simulink model "quartercar"  (R2013a)
settings: Solver=ode15s  StartTime=0  StopTime=60  RelTol=1e-3
libraries: simulink x3
settings Model: Creator=Administrator  LastModifiedBy=Tran Duc Chung
settings DataIOCC: LimitDataPoints=off

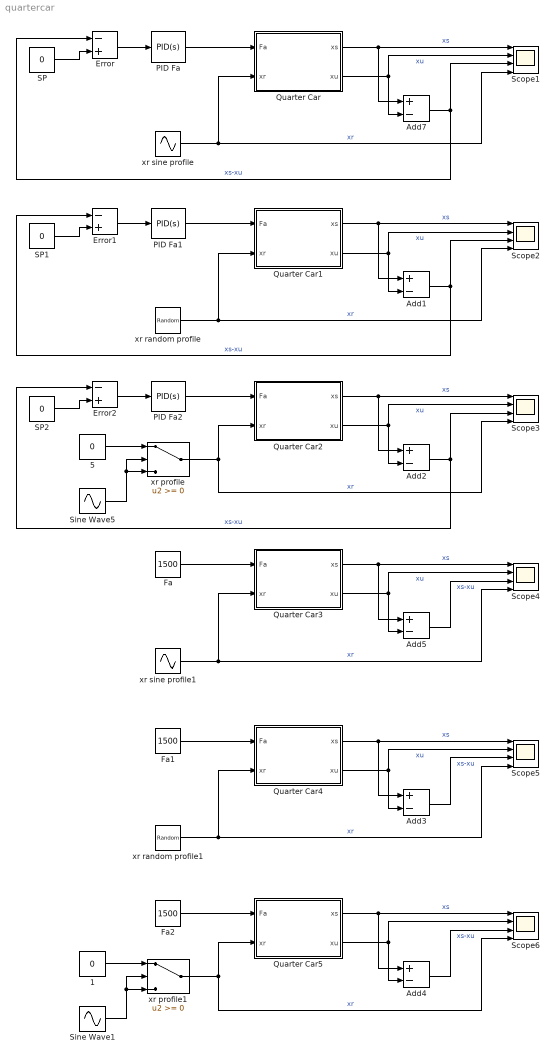
== system quartercar ==
  1 : Constant  Value=0
  5 : Constant  Value=0
  Add{1..5,7} (6 alike) : Sum  Inputs=+-
  Error : Sum  Inputs=-+
  Error1 : Sum  Inputs=-+
  Error2 : Sum  Inputs=-+
  Fa : Constant  Value=1500
  Fa1 : Constant  Value=1500
  Fa2 : Constant  Value=1500
  PID Fa : simulink/Continuous/PID Controller  Controller=PID  TimeDomain=Continuous-time  SampleTime=1  IntegratorMethod=Forward Euler  FilterMethod=Forward Euler  Form=Parallel  P=0  I=17490.1289315124  D=0  N=100  InitialConditionSource=internal  InitialConditionForIntegrator=0  InitialConditionForFilter=0  ExternalReset=none  LimitOutput=on  UpperSaturationLimit=3000  LowerSaturationLimit=0  LinearizeAsGain=on  AntiWindupMode=none  Kb=1  TrackingMode=off  Kt=1  PParamMin=[]  PParamMax=[]  IParamMin=[]  IParamMax=[]  DParamMin=[]  DParamMax=[]  NParamMin=[]  NParamMax=[]  KbParamMin=[]  KbParamMax=[]  KtParamMin=[]  KtParamMax=[]  POutMin=[]  POutMax=[]  IOutMin=[]  IOutMax=[]  DOutMin=[]  DOutMax=[]  NOutMin=[]  NOutMax=[]  KbOutMin=[]  KbOutMax=[]  KtOutMin=[]  KtOutMax=[]  IntegratorOutMin=[]  IntegratorOutMax=[]  FilterOutMin=[]  FilterOutMax=[]  SumOutMin=[]  SumOutMax=[]  SumI1OutMin=[]  SumI1OutMax=[]  SumI2OutMin=[]  SumI2OutMax=[]  SumI3OutMin=[]  SumI3OutMax=[]  SumDOutMin=[]  SumDOutMax=[]  SaturationOutMin=[]  SaturationOutMax=[]  IntegratorContinuousStateAttributes=''  IntegratorStateMustResolveToSignalObject=off  IntegratorRTWStateStorageClass=Auto  FilterContinuousStateAttributes=''  FilterStateMustResolveToSignalObject=off  FilterRTWStateStorageClass=Auto
  PID Fa1 : simulink/Continuous/PID Controller  Controller=PID  TimeDomain=Continuous-time  SampleTime=1  IntegratorMethod=Forward Euler  FilterMethod=Forward Euler  Form=Parallel  P=0  I=17490.1289315124  D=0  N=100  InitialConditionSource=internal  InitialConditionForIntegrator=0  InitialConditionForFilter=0  ExternalReset=none  LimitOutput=on  UpperSaturationLimit=3000  LowerSaturationLimit=0  LinearizeAsGain=on  AntiWindupMode=none  Kb=1  TrackingMode=off  Kt=1  PParamMin=[]  PParamMax=[]  IParamMin=[]  IParamMax=[]  DParamMin=[]  DParamMax=[]  NParamMin=[]  NParamMax=[]  KbParamMin=[]  KbParamMax=[]  KtParamMin=[]  KtParamMax=[]  POutMin=[]  POutMax=[]  IOutMin=[]  IOutMax=[]  DOutMin=[]  DOutMax=[]  NOutMin=[]  NOutMax=[]  KbOutMin=[]  KbOutMax=[]  KtOutMin=[]  KtOutMax=[]  IntegratorOutMin=[]  IntegratorOutMax=[]  FilterOutMin=[]  FilterOutMax=[]  SumOutMin=[]  SumOutMax=[]  SumI1OutMin=[]  SumI1OutMax=[]  SumI2OutMin=[]  SumI2OutMax=[]  SumI3OutMin=[]  SumI3OutMax=[]  SumDOutMin=[]  SumDOutMax=[]  SaturationOutMin=[]  SaturationOutMax=[]  IntegratorContinuousStateAttributes=''  IntegratorStateMustResolveToSignalObject=off  IntegratorRTWStateStorageClass=Auto  FilterContinuousStateAttributes=''  FilterStateMustResolveToSignalObject=off  FilterRTWStateStorageClass=Auto
  PID Fa2 : simulink/Continuous/PID Controller  Controller=PID  TimeDomain=Continuous-time  SampleTime=1  IntegratorMethod=Forward Euler  FilterMethod=Forward Euler  Form=Parallel  P=0  I=17490.1289315124  D=0  N=100  InitialConditionSource=internal  InitialConditionForIntegrator=0  InitialConditionForFilter=0  ExternalReset=none  LimitOutput=on  UpperSaturationLimit=3000  LowerSaturationLimit=0  LinearizeAsGain=on  AntiWindupMode=none  Kb=1  TrackingMode=off  Kt=1  PParamMin=[]  PParamMax=[]  IParamMin=[]  IParamMax=[]  DParamMin=[]  DParamMax=[]  NParamMin=[]  NParamMax=[]  KbParamMin=[]  KbParamMax=[]  KtParamMin=[]  KtParamMax=[]  POutMin=[]  POutMax=[]  IOutMin=[]  IOutMax=[]  DOutMin=[]  DOutMax=[]  NOutMin=[]  NOutMax=[]  KbOutMin=[]  KbOutMax=[]  KtOutMin=[]  KtOutMax=[]  IntegratorOutMin=[]  IntegratorOutMax=[]  FilterOutMin=[]  FilterOutMax=[]  SumOutMin=[]  SumOutMax=[]  SumI1OutMin=[]  SumI1OutMax=[]  SumI2OutMin=[]  SumI2OutMax=[]  SumI3OutMin=[]  SumI3OutMax=[]  SumDOutMin=[]  SumDOutMax=[]  SaturationOutMin=[]  SaturationOutMax=[]  IntegratorContinuousStateAttributes=''  IntegratorStateMustResolveToSignalObject=off  IntegratorRTWStateStorageClass=Auto  FilterContinuousStateAttributes=''  FilterStateMustResolveToSignalObject=off  FilterRTWStateStorageClass=Auto
  Quarter Car : Subsystem
  Quarter Car1 : Subsystem
  Quarter Car2 : Subsystem
  Quarter Car3 : Subsystem
  Quarter Car4 : Subsystem
  Quarter Car5 : Subsystem
  SP : Constant  Value=0
  SP1 : Constant  Value=0
  SP2 : Constant  Value=0
  Scope{1..6} (6 alike) : Scope  NumInputPorts=4
      Scope1 settings: YMin=-5~-5~-5~-5  YMax=5~5~5~5  SaveName=ScopeData3
      Scope2 settings: YMin=-5~-5~-5~-5  YMax=5~5~5~5
      Scope3 settings: YMin=-5~-5~-5~-5  YMax=5~5~5~5
      Scope4 settings: YMin=-5~-5~-5~-5  YMax=5~5~5~5  SaveName=ScopeData2
      Scope5 settings: YMin=-5~-5~-5~-5  YMax=5~5~5~5  SaveName=ScopeData4
      Scope6 settings: YMin=-5~-5~-5~-5  YMax=5~5~5~5  SaveName=ScopeData5
  Sine Wave1 : Sin  Amplitude=0.05  SampleTime=0
  Sine Wave5 : Sin  Amplitude=0.05  SampleTime=0
  xr profile : Switch
  xr profile1 : Switch
  xr random profile : RandomNumber  Variance=0.0005  SampleTime=0.1
  xr random profile1 : RandomNumber  Variance=0.0005  SampleTime=0.1
  xr sine profile : Sin  Amplitude=0.05  SampleTime=0
  xr sine profile1 : Sin  Amplitude=0.05  SampleTime=0
  wires:
  Error/1 -> PID Fa/1
  SP/1 -> Error/2
  5/1 -> xr profile/1
  Sine Wave5/1 -> xr profile/3, xr profile/2
  Quarter Car/1(xs) -> Add7/1, Scope1/1  "xs"
  Quarter Car/2(xu) -> Scope1/2, Add7/2  "xu"
  xr sine profile/1 -> Scope1/4, Quarter Car/2(xr)  "xr"
  PID Fa/1 -> Quarter Car/1(Fa)
  Add7/1 -> Scope1/3, Error/1  "xs-xu"
  Error1/1 -> PID Fa1/1
  SP1/1 -> Error1/2
  Quarter Car1/1(xs) -> Add1/1, Scope2/1  "xs"
  Quarter Car1/2(xu) -> Scope2/2, Add1/2  "xu"
  xr random profile/1 -> Scope2/4, Quarter Car1/2(xr)  "xr"
  PID Fa1/1 -> Quarter Car1/1(Fa)
  Add1/1 -> Scope2/3, Error1/1  "xs-xu"
  Error2/1 -> PID Fa2/1
  SP2/1 -> Error2/2
  Quarter Car2/1(xs) -> Add2/1, Scope3/1  "xs"
  Quarter Car2/2(xu) -> Scope3/2, Add2/2  "xu"
  xr profile/1 -> Scope3/4, Quarter Car2/2(xr)  "xr"
  PID Fa2/1 -> Quarter Car2/1(Fa)
  Add2/1 -> Scope3/3, Error2/1  "xs-xu"
  1/1 -> xr profile1/1
  Sine Wave1/1 -> xr profile1/3, xr profile1/2
  Quarter Car3/1(xs) -> Add5/1, Scope4/1  "xs"
  Quarter Car3/2(xu) -> Scope4/2, Add5/2  "xu"
  xr sine profile1/1 -> Scope4/4, Quarter Car3/2(xr)  "xr"
  Fa/1 -> Quarter Car3/1(Fa)
  Add5/1 -> Scope4/3  "xs-xu"
  Quarter Car4/1(xs) -> Add3/1, Scope5/1  "xs"
  Quarter Car4/2(xu) -> Scope5/2, Add3/2  "xu"
  xr random profile1/1 -> Scope5/4, Quarter Car4/2(xr)  "xr"
  Fa1/1 -> Quarter Car4/1(Fa)
  Add3/1 -> Scope5/3  "xs-xu"
  Quarter Car5/1(xs) -> Add4/1, Scope6/1  "xs"
  Quarter Car5/2(xu) -> Scope6/2, Add4/2
  xr profile1/1 -> Scope6/4, Quarter Car5/2(xr)  "xr"
  Fa2/1 -> Quarter Car5/1(Fa)
  Add4/1 -> Scope6/3  "xs-xu"

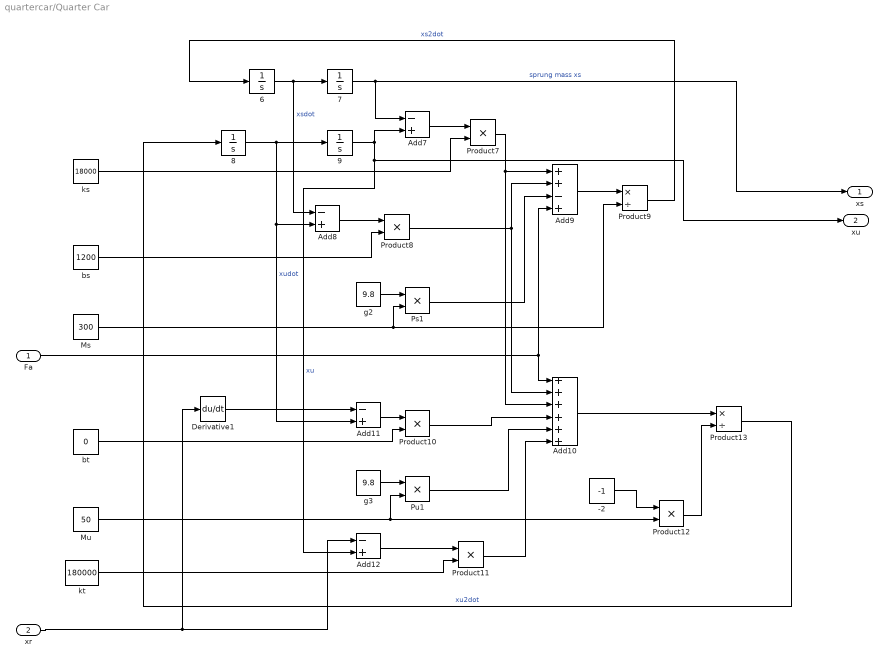
== system quartercar/Quarter Car ==
  Fa : Inport
  xr : Inport  Port=2
  -2 : Constant  Value=-1
  {6..9} (4 alike) : Integrator
  Add10 : Sum  Inputs=++++++
  Add{7..8,11..12} (4 alike) : Sum  Inputs=-+
  Add9 : Sum  Inputs=++-+
  Derivative1 : Derivative
  Ms : Constant  Value=300
  Mu : Constant  Value=50
  Product{7..8,10..12} (5 alike) : Product
  Product13 : Product  Inputs=*/
  Product9 : Product  Inputs=*/
  Ps1 : Product
  Pu1 : Product
  bs : Constant  Value=1200
  bt : Constant  Value=0
  g2 : Constant  Value=9.8
  g3 : Constant  Value=9.8
  ks : Constant  Value=18000
  kt : Constant  Value=180000
  xs : Outport
  xu : Outport  Port=2
  wires:
  g2/1 -> Ps1/1
  Product12/1 -> Product13/2
  g3/1 -> Pu1/1
  Ps1/1 -> Add9/3
  Add10/1 -> Product13/1
  -2/1 -> Product12/1
  Mu/1 -> Pu1/2, Product12/2
  Product11/1 -> Add10/6
  Add12/1 -> Product11/1
  kt/1 -> Product11/2
  xr/1 -> Add12/1, Derivative1/1
  Pu1/1 -> Add10/5
  Product10/1 -> Add10/4
  Add11/1 -> Product10/1
  bt/1 -> Product10/2
  Derivative1/1 -> Add11/1
  Ms/1 -> Product9/2, Ps1/2
  Add9/1 -> Product9/1
  Fa/1 -> Add10/1, Add9/4
  Product8/1 -> Add10/2, Add9/2
  Product7/1 -> Add10/3, Add9/1
  bs/1 -> Product8/2
  Add8/1 -> Product8/1
  ks/1 -> Product7/2
  Add7/1 -> Product7/1
  9/1 -> Add12/2, xu/1, Add7/2  "xu"
  Product13/1 -> 8/1  "xu2dot"
  8/1 -> 9/1, Add8/2, Add11/2  "xudot"
  7/1 -> Add7/1, xs/1  "sprung mass xs"
  Product9/1 -> 6/1  "xs2dot"
  6/1 -> 7/1, Add8/1  "xsdot"

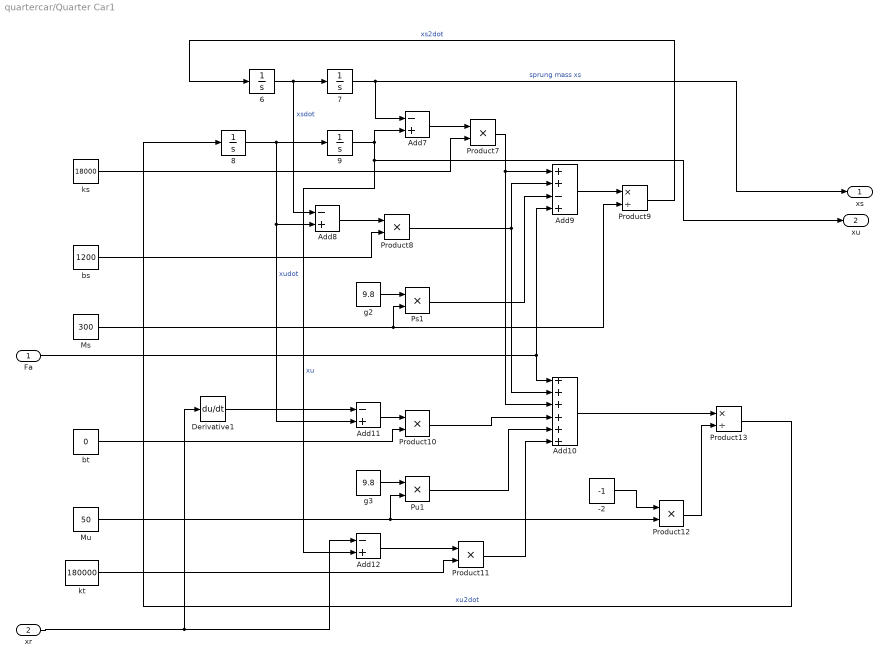
== system quartercar/Quarter Car1 ==
  Fa : Inport
  xr : Inport  Port=2
  -2 : Constant  Value=-1
  {6..9} (4 alike) : Integrator
  Add10 : Sum  Inputs=++++++
  Add{7..8,11..12} (4 alike) : Sum  Inputs=-+
  Add9 : Sum  Inputs=++-+
  Derivative1 : Derivative
  Ms : Constant  Value=300
  Mu : Constant  Value=50
  Product{7..8,10..12} (5 alike) : Product
  Product13 : Product  Inputs=*/
  Product9 : Product  Inputs=*/
  Ps1 : Product
  Pu1 : Product
  bs : Constant  Value=1200
  bt : Constant  Value=0
  g2 : Constant  Value=9.8
  g3 : Constant  Value=9.8
  ks : Constant  Value=18000
  kt : Constant  Value=180000
  xs : Outport
  xu : Outport  Port=2
  wires:
  g2/1 -> Ps1/1
  Product12/1 -> Product13/2
  g3/1 -> Pu1/1
  Ps1/1 -> Add9/3
  Add10/1 -> Product13/1
  -2/1 -> Product12/1
  Mu/1 -> Pu1/2, Product12/2
  Product11/1 -> Add10/6
  Add12/1 -> Product11/1
  kt/1 -> Product11/2
  xr/1 -> Add12/1, Derivative1/1
  Pu1/1 -> Add10/5
  Product10/1 -> Add10/4
  Add11/1 -> Product10/1
  bt/1 -> Product10/2
  Derivative1/1 -> Add11/1
  Ms/1 -> Product9/2, Ps1/2
  Add9/1 -> Product9/1
  Fa/1 -> Add10/1, Add9/4
  Product8/1 -> Add10/2, Add9/2
  Product7/1 -> Add10/3, Add9/1
  bs/1 -> Product8/2
  Add8/1 -> Product8/1
  ks/1 -> Product7/2
  Add7/1 -> Product7/1
  9/1 -> Add12/2, xu/1, Add7/2  "xu"
  Product13/1 -> 8/1  "xu2dot"
  8/1 -> 9/1, Add8/2, Add11/2  "xudot"
  7/1 -> Add7/1, xs/1  "sprung mass xs"
  Product9/1 -> 6/1  "xs2dot"
  6/1 -> 7/1, Add8/1  "xsdot"

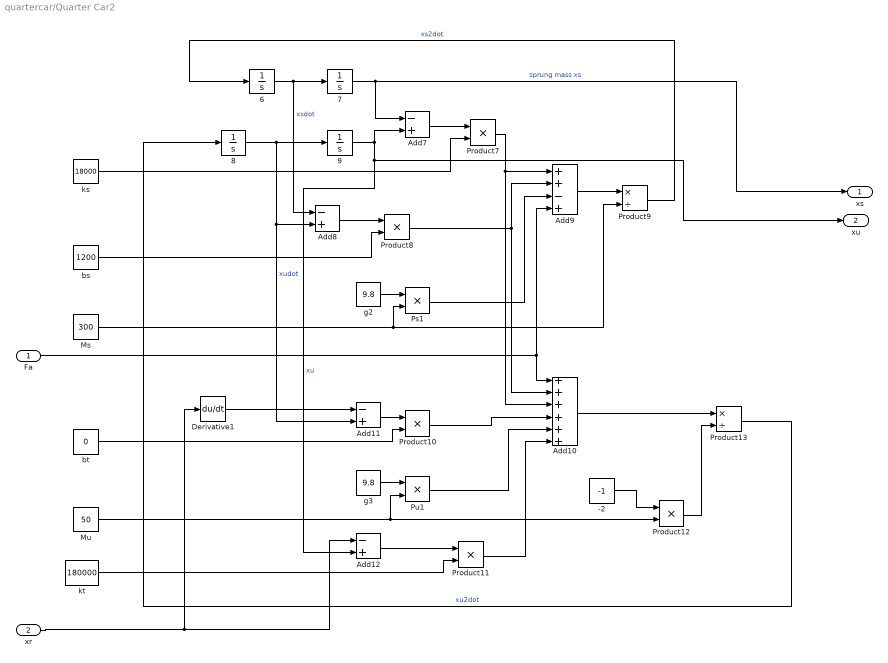
== system quartercar/Quarter Car2 ==
  Fa : Inport
  xr : Inport  Port=2
  -2 : Constant  Value=-1
  {6..9} (4 alike) : Integrator
  Add10 : Sum  Inputs=++++++
  Add{7..8,11..12} (4 alike) : Sum  Inputs=-+
  Add9 : Sum  Inputs=++-+
  Derivative1 : Derivative
  Ms : Constant  Value=300
  Mu : Constant  Value=50
  Product{7..8,10..12} (5 alike) : Product
  Product13 : Product  Inputs=*/
  Product9 : Product  Inputs=*/
  Ps1 : Product
  Pu1 : Product
  bs : Constant  Value=1200
  bt : Constant  Value=0
  g2 : Constant  Value=9.8
  g3 : Constant  Value=9.8
  ks : Constant  Value=18000
  kt : Constant  Value=180000
  xs : Outport
  xu : Outport  Port=2
  wires:
  g2/1 -> Ps1/1
  Product12/1 -> Product13/2
  g3/1 -> Pu1/1
  Ps1/1 -> Add9/3
  Add10/1 -> Product13/1
  -2/1 -> Product12/1
  Mu/1 -> Pu1/2, Product12/2
  Product11/1 -> Add10/6
  Add12/1 -> Product11/1
  kt/1 -> Product11/2
  xr/1 -> Add12/1, Derivative1/1
  Pu1/1 -> Add10/5
  Product10/1 -> Add10/4
  Add11/1 -> Product10/1
  bt/1 -> Product10/2
  Derivative1/1 -> Add11/1
  Ms/1 -> Product9/2, Ps1/2
  Add9/1 -> Product9/1
  Fa/1 -> Add10/1, Add9/4
  Product8/1 -> Add10/2, Add9/2
  Product7/1 -> Add10/3, Add9/1
  bs/1 -> Product8/2
  Add8/1 -> Product8/1
  ks/1 -> Product7/2
  Add7/1 -> Product7/1
  9/1 -> Add12/2, xu/1, Add7/2  "xu"
  Product13/1 -> 8/1  "xu2dot"
  8/1 -> 9/1, Add8/2, Add11/2  "xudot"
  7/1 -> Add7/1, xs/1  "sprung mass xs"
  Product9/1 -> 6/1  "xs2dot"
  6/1 -> 7/1, Add8/1  "xsdot"

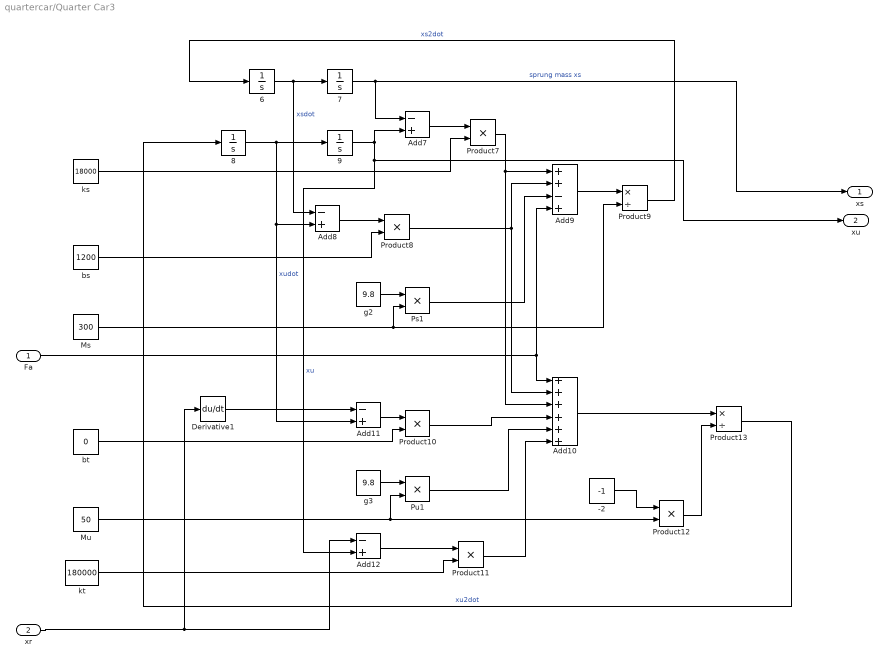
== system quartercar/Quarter Car3 ==
  Fa : Inport
  xr : Inport  Port=2
  -2 : Constant  Value=-1
  {6..9} (4 alike) : Integrator
  Add10 : Sum  Inputs=++++++
  Add{7..8,11..12} (4 alike) : Sum  Inputs=-+
  Add9 : Sum  Inputs=++-+
  Derivative1 : Derivative
  Ms : Constant  Value=300
  Mu : Constant  Value=50
  Product{7..8,10..12} (5 alike) : Product
  Product13 : Product  Inputs=*/
  Product9 : Product  Inputs=*/
  Ps1 : Product
  Pu1 : Product
  bs : Constant  Value=1200
  bt : Constant  Value=0
  g2 : Constant  Value=9.8
  g3 : Constant  Value=9.8
  ks : Constant  Value=18000
  kt : Constant  Value=180000
  xs : Outport
  xu : Outport  Port=2
  wires:
  g2/1 -> Ps1/1
  Product12/1 -> Product13/2
  g3/1 -> Pu1/1
  Ps1/1 -> Add9/3
  Add10/1 -> Product13/1
  -2/1 -> Product12/1
  Mu/1 -> Pu1/2, Product12/2
  Product11/1 -> Add10/6
  Add12/1 -> Product11/1
  kt/1 -> Product11/2
  xr/1 -> Add12/1, Derivative1/1
  Pu1/1 -> Add10/5
  Product10/1 -> Add10/4
  Add11/1 -> Product10/1
  bt/1 -> Product10/2
  Derivative1/1 -> Add11/1
  Ms/1 -> Product9/2, Ps1/2
  Add9/1 -> Product9/1
  Fa/1 -> Add10/1, Add9/4
  Product8/1 -> Add10/2, Add9/2
  Product7/1 -> Add10/3, Add9/1
  bs/1 -> Product8/2
  Add8/1 -> Product8/1
  ks/1 -> Product7/2
  Add7/1 -> Product7/1
  9/1 -> Add12/2, xu/1, Add7/2  "xu"
  Product13/1 -> 8/1  "xu2dot"
  8/1 -> 9/1, Add8/2, Add11/2  "xudot"
  7/1 -> Add7/1, xs/1  "sprung mass xs"
  Product9/1 -> 6/1  "xs2dot"
  6/1 -> 7/1, Add8/1  "xsdot"

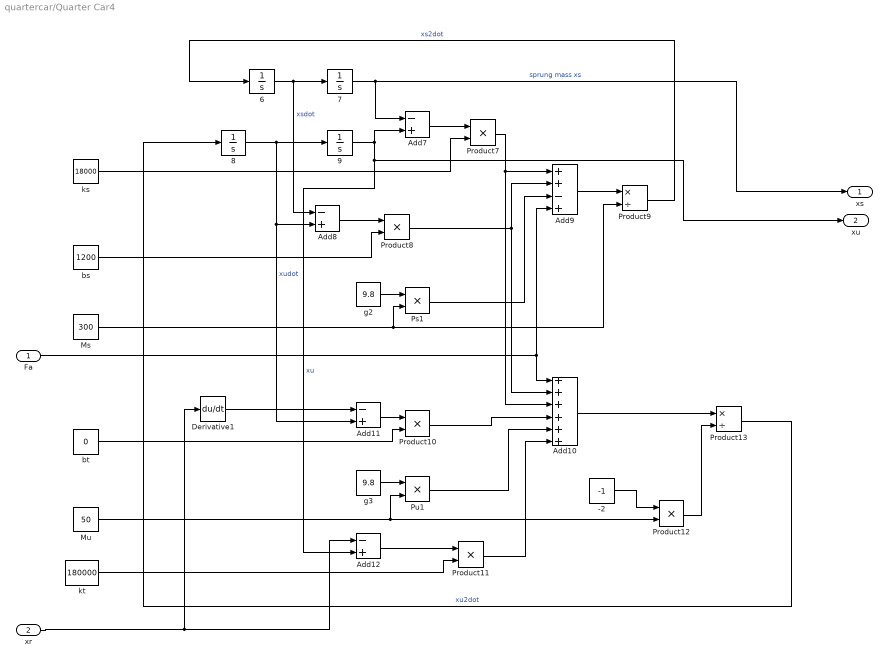
== system quartercar/Quarter Car4 ==
  Fa : Inport
  xr : Inport  Port=2
  -2 : Constant  Value=-1
  {6..9} (4 alike) : Integrator
  Add10 : Sum  Inputs=++++++
  Add{7..8,11..12} (4 alike) : Sum  Inputs=-+
  Add9 : Sum  Inputs=++-+
  Derivative1 : Derivative
  Ms : Constant  Value=300
  Mu : Constant  Value=50
  Product{7..8,10..12} (5 alike) : Product
  Product13 : Product  Inputs=*/
  Product9 : Product  Inputs=*/
  Ps1 : Product
  Pu1 : Product
  bs : Constant  Value=1200
  bt : Constant  Value=0
  g2 : Constant  Value=9.8
  g3 : Constant  Value=9.8
  ks : Constant  Value=18000
  kt : Constant  Value=180000
  xs : Outport
  xu : Outport  Port=2
  wires:
  g2/1 -> Ps1/1
  Product12/1 -> Product13/2
  g3/1 -> Pu1/1
  Ps1/1 -> Add9/3
  Add10/1 -> Product13/1
  -2/1 -> Product12/1
  Mu/1 -> Pu1/2, Product12/2
  Product11/1 -> Add10/6
  Add12/1 -> Product11/1
  kt/1 -> Product11/2
  xr/1 -> Add12/1, Derivative1/1
  Pu1/1 -> Add10/5
  Product10/1 -> Add10/4
  Add11/1 -> Product10/1
  bt/1 -> Product10/2
  Derivative1/1 -> Add11/1
  Ms/1 -> Product9/2, Ps1/2
  Add9/1 -> Product9/1
  Fa/1 -> Add10/1, Add9/4
  Product8/1 -> Add10/2, Add9/2
  Product7/1 -> Add10/3, Add9/1
  bs/1 -> Product8/2
  Add8/1 -> Product8/1
  ks/1 -> Product7/2
  Add7/1 -> Product7/1
  9/1 -> Add12/2, xu/1, Add7/2  "xu"
  Product13/1 -> 8/1  "xu2dot"
  8/1 -> 9/1, Add8/2, Add11/2  "xudot"
  7/1 -> Add7/1, xs/1  "sprung mass xs"
  Product9/1 -> 6/1  "xs2dot"
  6/1 -> 7/1, Add8/1  "xsdot"

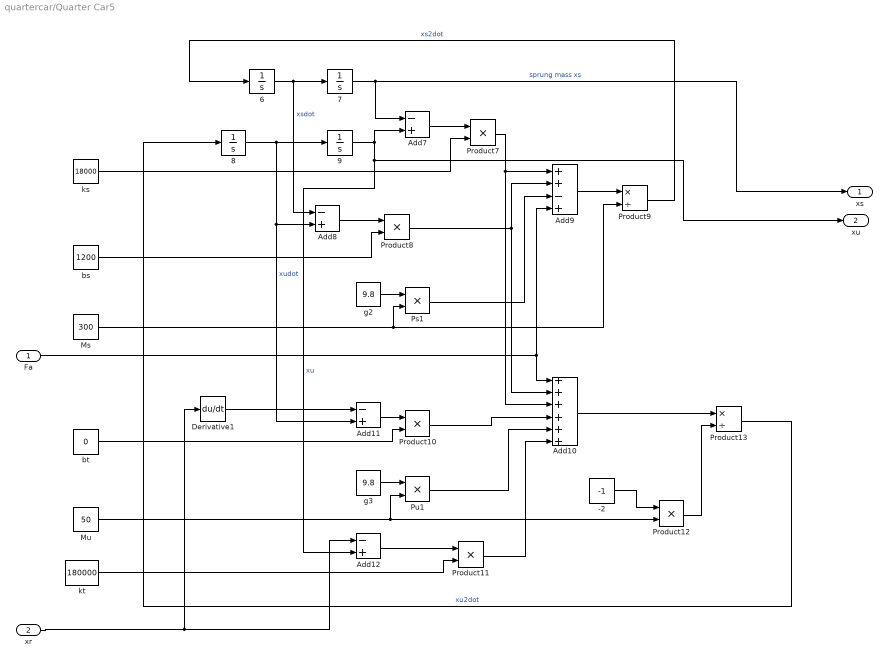
== system quartercar/Quarter Car5 ==
  Fa : Inport
  xr : Inport  Port=2
  -2 : Constant  Value=-1
  {6..9} (4 alike) : Integrator
  Add10 : Sum  Inputs=++++++
  Add{7..8,11..12} (4 alike) : Sum  Inputs=-+
  Add9 : Sum  Inputs=++-+
  Derivative1 : Derivative
  Ms : Constant  Value=300
  Mu : Constant  Value=50
  Product{7..8,10..12} (5 alike) : Product
  Product13 : Product  Inputs=*/
  Product9 : Product  Inputs=*/
  Ps1 : Product
  Pu1 : Product
  bs : Constant  Value=1200
  bt : Constant  Value=0
  g2 : Constant  Value=9.8
  g3 : Constant  Value=9.8
  ks : Constant  Value=18000
  kt : Constant  Value=180000
  xs : Outport
  xu : Outport  Port=2
  wires:
  g2/1 -> Ps1/1
  Product12/1 -> Product13/2
  g3/1 -> Pu1/1
  Ps1/1 -> Add9/3
  Add10/1 -> Product13/1
  -2/1 -> Product12/1
  Mu/1 -> Pu1/2, Product12/2
  Product11/1 -> Add10/6
  Add12/1 -> Product11/1
  kt/1 -> Product11/2
  xr/1 -> Add12/1, Derivative1/1
  Pu1/1 -> Add10/5
  Product10/1 -> Add10/4
  Add11/1 -> Product10/1
  bt/1 -> Product10/2
  Derivative1/1 -> Add11/1
  Ms/1 -> Product9/2, Ps1/2
  Add9/1 -> Product9/1
  Fa/1 -> Add10/1, Add9/4
  Product8/1 -> Add10/2, Add9/2
  Product7/1 -> Add10/3, Add9/1
  bs/1 -> Product8/2
  Add8/1 -> Product8/1
  ks/1 -> Product7/2
  Add7/1 -> Product7/1
  9/1 -> Add12/2, xu/1, Add7/2  "xu"
  Product13/1 -> 8/1  "xu2dot"
  8/1 -> 9/1, Add8/2, Add11/2  "xudot"
  7/1 -> Add7/1, xs/1  "sprung mass xs"
  Product9/1 -> 6/1  "xs2dot"
  6/1 -> 7/1, Add8/1  "xsdot"
